simulink model "EmbeddedCoder_CSE347"  (R2018a)
settings: Solver=VariableStepAuto  StartTime=0.0  StopTime=30  FixedStep=0.01  RelTol=1e-3
libraries: simulink_extras x2, simulink x1
settings Model: Creator=micha  LastModifiedBy=micha
settings OptimizationCC: DefaultParameterBehavior=Inlined  EnhancedBackFolding=on  PassReuseOutputArgsAs=Individual arguments  OptimizeBlockOrder=speed  DifferentSizesBufferReuse=on
settings DebuggingCC: ParameterTunabilityLossMsg=error
settings SFSimCC: MATLABDynamicMemAlloc=off
settings RTWCC: SystemTargetFile=ert.tlc  TemplateMakefile=ert_default_tmf  GenerateReport=on  IncludeHyperlinkInReport=on  LaunchReport=on  GenerateTraceInfo=on  GenerateTraceReport=on  GenerateTraceReportSl=on  GenerateTraceReportSf=on  GenerateTraceReportEml=on
settings CodeAppCC: ForceParamTrailComments=on  IgnoreCustomStorageClasses=off  OperatorAnnotations=on  SimulinkDataObjDesc=on  SFDataObjDesc=on  InsertBlockDesc=on
settings ERTTargetCC: TargetLangStandard=C99 (ISO)  GenerateSampleERTMain=on  InlinedParameterPlacement=NonHierarchical  ERTCustomFileTemplate=example_file_process.tlc

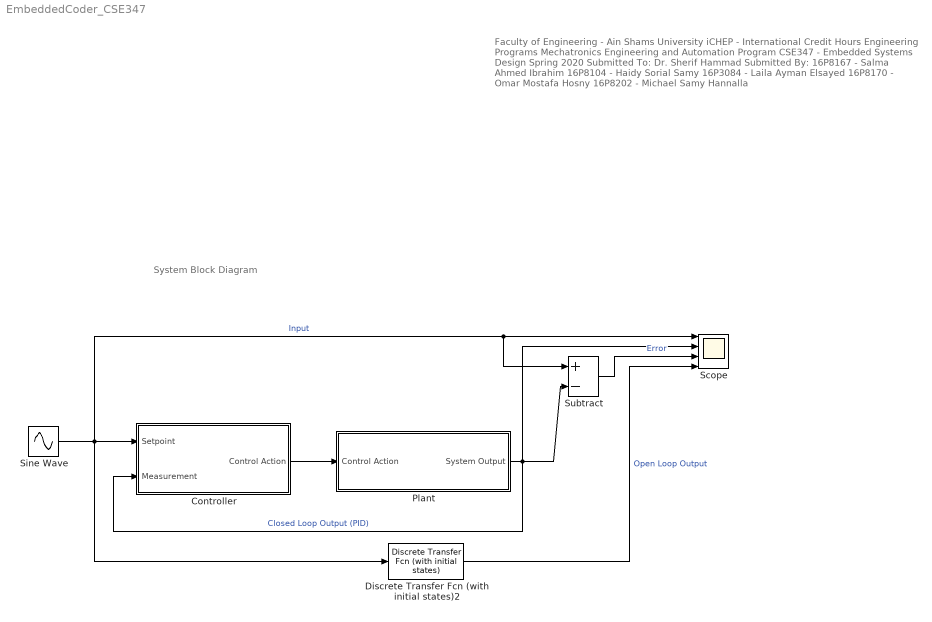
== system EmbeddedCoder_CSE347 ==
  note: Faculty of Engineering - Ain Shams University
      | iCHEP - International Credit Hours Engineering Programs
      | Mechatronics Engineering and Automation Program
      | CSE347 - Embedded Systems Design
      | Spring 2020
      |
      | Submitted To:
      | Dr. Sherif Hammad
      |
      | Submitted By:
      | 16P8167 - Salma Ahmed Ibrahim
      | 16P8104 - Haidy Sorial Samy
      | 16P3084 - Laila Ayman Elsayed
      | 16P8170 - Omar Mostafa Hosny
      | 16P8202 - Michael Samy Hannalla
  note: System Block Diagram
  Controller : Subsystem
  Discrete Transfer Fcn (with initial states)2 : simulink_extras/Additional Discrete/Discrete Transfer Fcn (with initial states)  N=[1]  D=[1 0.5]  X0=[0]  TS=.01
      settings: SourceProductName=Simulink  SourceProductBaseCode=SL
  Plant : Subsystem
  Scope : Scope  NumInputPorts=4
  Sine Wave : Sin  SampleTime=0.1
  Subtract : Sum  Inputs=+-  OutDataTypeStr=Inherit: Inherit via back propagation
  wires:
  Controller/1(Control Action) -> Plant/1(Control Action)
  Sine Wave/1 -> Discrete Transfer Fcn (with initial states)2/1, Subtract/1, Scope/1, Controller/1(Setpoint)  "Input"
  Plant/1(System Output) -> Subtract/2, Scope/2, Controller/2(Measurement)  "Closed Loop Output (PID)"
  Discrete Transfer Fcn (with initial states)2/1 -> Scope/4  "Open Loop Output"
  Subtract/1 -> Scope/3  "Error"

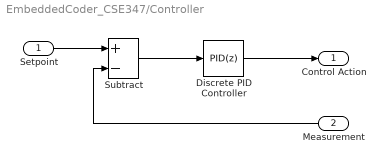
== system EmbeddedCoder_CSE347/Controller ==
  Setpoint : Inport
  Measurement : Inport  Port=2
  Discrete PID Controller : simulink/Continuous/PID Controller  Controller=PID  TimeDomain=Discrete-time  SampleTime=-1  IntegratorMethod=Forward Euler  FilterMethod=Forward Euler  Form=Parallel  UseFilter=on  ControllerParametersSource=internal  P=0.0074999791668287  I=1.49999583336574  D=0  N=100  InitialConditionSource=internal  InitialConditionForIntegrator=0  InitialConditionForFilter=0  ExternalReset=none  LimitOutput=off  UpperSaturationLimit=inf  LowerSaturationLimit=-inf  LinearizeAsGain=off  AntiWindupMode=none  Kb=1  TrackingMode=off  Kt=1  PParamMin=[]  PParamMax=[]  IParamMin=[]  IParamMax=[]  DParamMin=[]  DParamMax=[]  NParamMin=[]  NParamMax=[]  KbParamMin=[]  KbParamMax=[]  KtParamMin=[]  KtParamMax=[]  POutMin=[]  POutMax=[]  IOutMin=[]  IOutMax=[]  DOutMin=[]  DOutMax=[]  NOutMin=[]  NOutMax=[]  KbOutMin=[]  KbOutMax=[]  KtOutMin=[]  KtOutMax=[]  IntegratorOutMin=[]  IntegratorOutMax=[]  FilterOutMin=[]  FilterOutMax=[]  SumOutMin=[]  SumOutMax=[]  SumI1OutMin=[]  SumI1OutMax=[]  SumI2OutMin=[]  SumI2OutMax=[]  SumI3OutMin=[]  SumI3OutMax=[]  SumDOutMin=[]  SumDOutMax=[]  SaturationOutMin=[]  SaturationOutMax=[]  IntegratorContinuousStateAttributes=''  IntegratorStateMustResolveToSignalObject=off  IntegratorRTWStateStorageClass=Auto  FilterContinuousStateAttributes=''  FilterStateMustResolveToSignalObject=off  FilterRTWStateStorageClass=Auto  DifferentiatorICPrevScaledInput=0  DifferentiatorOutMin=[]  DifferentiatorOutMax=[]  FilterDiffOutCoefMin=[]  FilterDiffOutCoefMax=[]  SumDenOutMin=[]  SumDenOutMax=[]  SumNumOutMin=[]  SumNumOutMax=[]  ReciprocalOutMin=[]  ReciprocalOutMax=[]  DivideOutMin=[]  DivideOutMax=[]  TunerSelectOption=Transfer Function Based (PID Tuner App)
  Subtract : Sum  Inputs=+-  OutDataTypeStr=Inherit: Inherit via back propagation
  Control Action : Outport
  wires:
  Subtract/1 -> Discrete PID Controller/1
  Setpoint/1 -> Subtract/1
  Discrete PID Controller/1 -> Control Action/1
  Measurement/1 -> Subtract/2

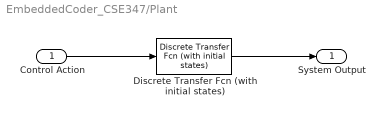
== system EmbeddedCoder_CSE347/Plant ==
  Control Action : Inport
  Discrete Transfer Fcn (with initial states) : simulink_extras/Additional Discrete/Discrete Transfer Fcn (with initial states)  N=[1]  D=[1 0.5]  X0=[0]  TS=.01
      settings: SourceProductName=Simulink  SourceProductBaseCode=SL
  System Output : Outport
  wires:
  Discrete Transfer Fcn (with initial states)/1 -> System Output/1
  Control Action/1 -> Discrete Transfer Fcn (with initial states)/1
